simulink model "SimFreqDynamics"  (R2023a)
settings: Solver=VariableStepAuto  StartTime=0.0  StopTime=0.4  RelTol=1e-3
values from neighbouring files (symbols this model uses):
  L = X/Wbase    (= 0.0031194368846)    [ParaFreqVoltageEquivalance.m]
  R = X/5    (= 0.196)    [ParaFreqVoltageEquivalance.m]
  Sbase = 1    [ParaFreqDynamics.m]    (also in ParaFreqVoltageEquivalance.m; SimModel_Parameters.m)
  Ts = 1/Fs    (= 1e-05)    [ParaFreqDynamics.m]    (also in ParaFreqVoltageEquivalance.m; SimModel_Parameters.m = 0.0001)
  Vbase = 1    [ParaFreqDynamics.m]    (also in ParaFreqVoltageEquivalance.m; SimModel_Parameters.m)
  Wbase = Fbase*2*pi    (= 314.159265359)    [ParaFreqDynamics.m]    (also in ParaFreqVoltageEquivalance.m; SimModel_Parameters.m)
undefined symbols (not defined in the file or in its folder): DiscIntNeverNeededParam
libraries: spsCurrentMeasurementLib x6, spsSeriesRLCBranchLib x3, spsControlledVoltageSourceLib x3, spsGroundLib x2, SimplusGT x1, spsThreePhaseSeriesRLCBranchLib x1, sps_lib x1
settings Model: Creator=admin_user  LastModifiedBy=admin_user

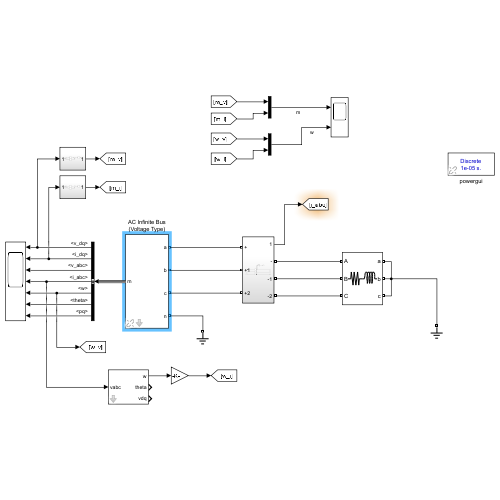
[thumbnail: Simulink's stored preview of the top-level diagram]
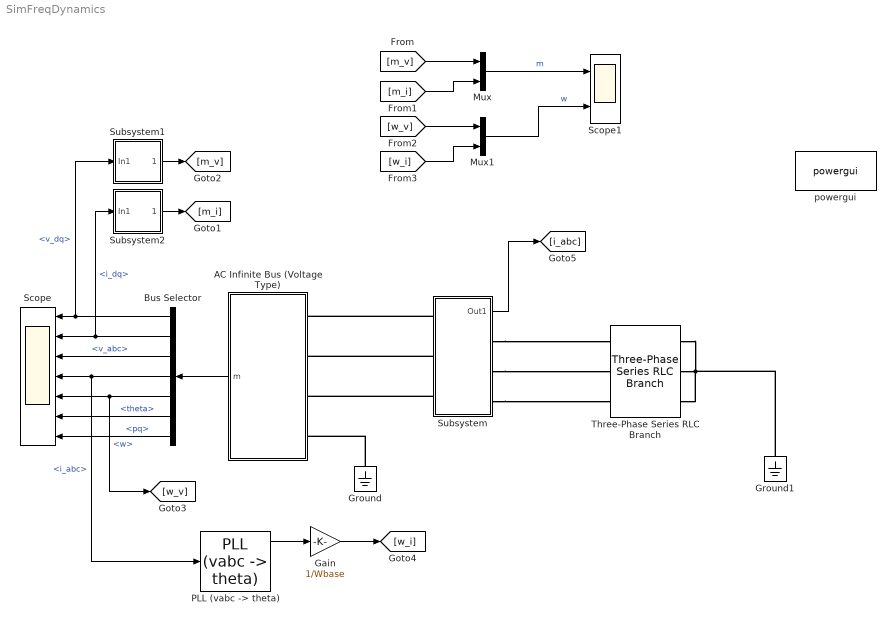
== system SimFreqDynamics ==
  AC Infinite Bus (Voltage Type) : Subsystem  AncestorBlock=|  mask{Ts=Ts, Sbase=Sbase, Vbase=Vbase, Wbase=Wbase, vd=1, vq=0, theta0=0, w=Wbase, R=1e-30}
      | SimplusGT/AC Infinite Bus
      | (Voltage Type)
      mask prompts: Ts "Ts (s), samping period"; Sbase "Sbase (VA), power base"; Vbase "Vbase (V), voltage base"; Wbase "Wbase (rad/s), frequency base"; vd "vd (pu), d-axis voltage"; vq "vq (pu), q-axis voltage"; theta0 "theta0 (rad), initial angle"; w "w (rad/s), frequency"; R "R (Ohm), resistance"
  Bus Selector : BusSelector  OutputSignals=v_dq,i_dq,v_abc,i_abc,w,theta,pq
  Gain : Gain  Gain=1/Wbase
  Ground : spsGroundLib/Ground  LConnTagsString=a
  Ground1 : spsGroundLib/Ground  LConnTagsString=a
  Mux : Mux  Inputs=2
  Mux1 : Mux  Inputs=2
  "PLL (vabc -> theta)" : SimplusGT/PLL (vabc -> theta)  Ts=Ts  Wbase=Wbase  w_pll=w_pll  w_tau=w_tau  theta0=0
      settings: SourceProductName=Simplus Grid Tool
  Scope : Scope  NumInputPorts=7
  Scope1 : Scope  NumInputPorts=2
  Subsystem : Subsystem
  Subsystem1 : Subsystem
  Subsystem2 : Subsystem
  Three-Phase Series RLC Branch : spsThreePhaseSeriesRLCBranchLib/Three-Phase Series RLC Branch  LConnTagsString=A|B|C  RConnTagsString=A|B|C  BranchType=RL  Resistance=R  Inductance=L  Capacitance=1e-6  Measurements=None
  powergui : sps_lib/powergui  Priority=1  SimulationMode=Discrete  SampleTime=Ts  frequency=60  Iterations=50  frequencyindice=0  Pbase=100e6  ErrMax=1e-4  UnitsV=kV  UnitsW=MW  buscounter=0  FunctionMessages=off  echomessages=off  EnableUseOfTLC=off  CurrentSourceSwitches=off  DisableSnubberDevices=off  DisableRonSwitches=off  DisableVfSwitches=off  DisplayEquations=off  AutomaticDiscreteSolvers=off  SolverType=Tustin/Backward Euler (TBE)  Interpol=off  ExternalGateDelay=off  methode=off  Ts=100  x0status=blocks  SPID=on  SwTol=0  HookPort=off  NonlinearTolerance=1e-4  nMaxIteration=100  ContinueOnMaxIteration=off  RestoreLinks=warning  ResistiveCurrentMeasurement=off  Frange=[0:2:500]  Ylog=off  Xlog=on  ShowGrid=off  save=off  variable=ZData  structure=0  ZoomFFT=off  StartTime=0.0  cycles=1  DisplayStyle=1  fundamental=60  FreqAxis=off  MaxFrequency=1000  frequencyindicesteady=1  RmsSteady=1  display=off
  wires:
  AC Infinite Bus (Voltage Type)/1(m) -> Bus Selector/1
  Bus Selector/1 -> Subsystem1/1(In1), Scope/1  "<v_dq>"
  Bus Selector/3 -> Scope/3  "<v_abc>"
  Bus Selector/4 -> "PLL (vabc -> theta)"/1, Scope/4  "<i_abc>"
  Bus Selector/5 -> [w_v], Scope/5  "<w>"
  Bus Selector/6 -> Scope/6  "<theta>"
  Bus Selector/7 -> Scope/7  "<pq>"
  Subsystem/1(Out1) -> [i_abc]
  Subsystem1/1(Out1) -> [m_v]
  Bus Selector/2 -> Scope/2, Subsystem2/1(In1)  "<i_dq>"
  Subsystem2/1(Out1) -> [m_i]
  "PLL (vabc -> theta)"/1 -> Gain/1
  [m_v] -> Mux/1
  [m_i] -> Mux/2
  [w_v] -> Mux1/1
  [w_i] -> Mux1/2
  Mux/1 -> Scope1/1  "m"
  Mux1/1 -> Scope1/2  "w"
  Gain/1 -> [w_i]
  connections:
  Three-Phase Series RLC Branch/RConn1 -- Three-Phase Series RLC Branch/RConn2 -- Three-Phase Series RLC Branch/RConn3 -- Ground1/LConn1
  Ground/LConn1 -- AC Infinite Bus (Voltage Type)/LConn4
  Subsystem/LConn1 -- AC Infinite Bus (Voltage Type)/LConn1
  Subsystem/RConn1 -- Three-Phase Series RLC Branch/LConn1
  Subsystem/LConn2 -- AC Infinite Bus (Voltage Type)/LConn2
  Subsystem/RConn2 -- Three-Phase Series RLC Branch/LConn2
  Subsystem/LConn3 -- AC Infinite Bus (Voltage Type)/LConn3
  Subsystem/RConn3 -- Three-Phase Series RLC Branch/LConn3

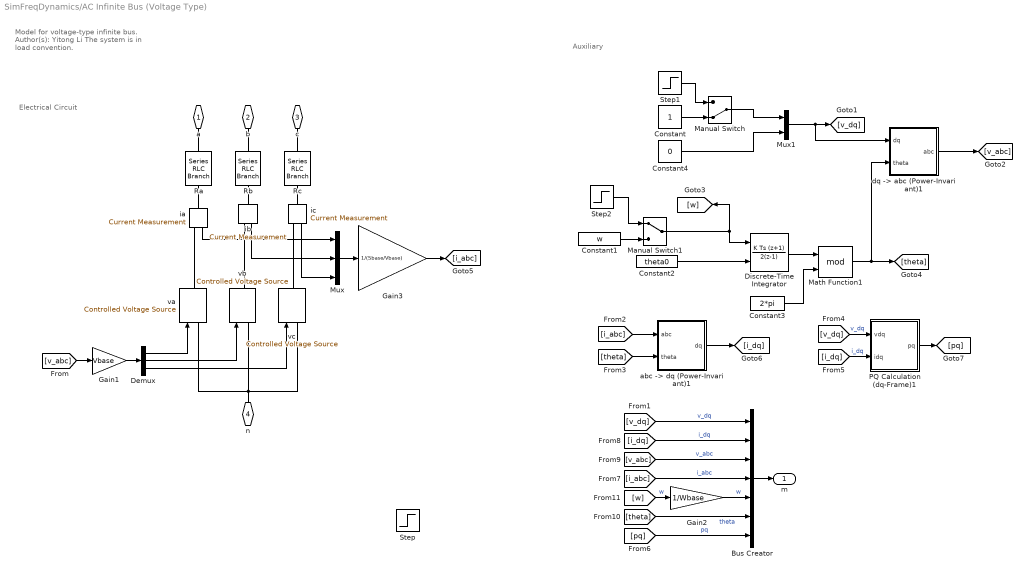
== system SimFreqDynamics/AC Infinite Bus (Voltage Type) ==
  note: Auxiliary
  note: Electrical Circuit
  note: Model for voltage-type infinite bus.
      |
      | Author(s): Yitong Li
      |
      | The system is in load convention.
  Bus Creator : BusCreator  Inputs=7
  Constant : Constant
  Constant1 : Constant  Value=w
  Constant2 : Constant  Value=theta0
  Constant3 : Constant  Value=2*pi
  Constant4 : Constant  Value=0
  Demux : Demux  Outputs=3
  Discrete-Time Integrator : DiscreteIntegrator  IntegratorMethod=Integration: Trapezoidal  InitialConditionSource=external  SampleTime=-1  ICPrevOutput=DiscIntNeverNeededParam  ICPrevScaledInput=DiscIntNeverNeededParam
  Gain1 : Gain  Gain=Vbase
  Gain2 : Gain  Gain=1/Wbase
  Gain3 : Gain  Gain=1/(Sbase/Vbase)
  Manual Switch : ManualSwitch  CurrentSetting=0
  Manual Switch1 : ManualSwitch
  Math Function1 : Math  Operator=mod  SignedPower=on
  Mux : Mux  Inputs=3
  Mux1 : Mux  Inputs=2
  PQ Calculation (dq-Frame)1 : Subsystem  AncestorBlock=|
      | SimplusGT/PQ Calculation
      | (dq-Frame)
  Ra : spsSeriesRLCBranchLib/Series RLC Branch  LConnTagsString=__new0  RConnTagsString=__new0  BranchType=R  Resistance=R  Inductance=1e-3  SetiL0=off  InitialCurrent=0  Capacitance=1e-6  Setx0=off  InitialVoltage=0  Measurements=None
  Rb : spsSeriesRLCBranchLib/Series RLC Branch  LConnTagsString=__new0  RConnTagsString=__new0  BranchType=R  Resistance=R  Inductance=1e-3  SetiL0=off  InitialCurrent=0  Capacitance=1e-6  Setx0=off  InitialVoltage=0  Measurements=None
  Rc : spsSeriesRLCBranchLib/Series RLC Branch  LConnTagsString=__new0  RConnTagsString=__new0  BranchType=R  Resistance=R  Inductance=1e-3  SetiL0=off  InitialCurrent=0  Capacitance=1e-6  Setx0=off  InitialVoltage=0  Measurements=None
  Step : Step  SampleTime=0
  Step1 : Step  Time=0.2  Before=1  After=1.1  SampleTime=0
  Step2 : Step  Time=0.2  Before=1*Wbase  After=1.1*Wbase  SampleTime=0
  "abc -> dq (Power-Invariant)1" : Subsystem  AncestorBlock=|
      | SimplusGT/abc -> dq
      | (Power-Invariant)
  "dq -> abc (Power-Invariant)1" : Subsystem  AncestorBlock=|
      | SimplusGT/dq -> abc
      | (Power-Invariant)
  ia : spsCurrentMeasurementLib/Current Measurement  PhasorSimulation=off  OutputType=Complex  PSBequivalent=0
  ib : spsCurrentMeasurementLib/Current Measurement  PhasorSimulation=off  OutputType=Complex  PSBequivalent=0
  ic : spsCurrentMeasurementLib/Current Measurement  PhasorSimulation=off  OutputType=Complex  PSBequivalent=0
  va : spsControlledVoltageSourceLib/Controlled Voltage Source  Initialize=on  Source_Type=AC  Amplitude=0  Phase=0  Frequency=0  Measurements=None
  vb : spsControlledVoltageSourceLib/Controlled Voltage Source  Initialize=on  Source_Type=AC  Amplitude=0  Phase=0  Frequency=0  Measurements=None
  vc : spsControlledVoltageSourceLib/Controlled Voltage Source  Initialize=on  Source_Type=AC  Amplitude=0  Phase=0  Frequency=0  Measurements=None
  a : PMIOPort  Side=Left
  b : PMIOPort  Port=2  Side=Left
  c : PMIOPort  Port=3  Side=Left
  n : PMIOPort  Port=4  Side=Left
  m : Outport
  wires:
  [pq] -> Bus Creator/7  "pq"
  PQ Calculation (dq-Frame)1/1(pq) -> [pq]
  [i_dq] -> PQ Calculation (dq-Frame)1/2(idq)  "i_dq"
  [v_dq] -> PQ Calculation (dq-Frame)1/1(vdq)  "v_dq"
  Gain3/1 -> [i_abc]
  Mux/1 -> Gain3/1
  Gain1/1 -> Demux/1
  "abc -> dq (Power-Invariant)1"/1(dq) -> [i_dq]
  [theta] -> "abc -> dq (Power-Invariant)1"/2(theta)
  [i_abc] -> "abc -> dq (Power-Invariant)1"/1(abc)
  ic/1 -> Mux/3
  ib/1 -> Mux/2
  ia/1 -> Mux/1
  [theta] -> Bus Creator/6  "theta"
  Bus Creator/1 -> m/1
  [i_dq] -> Bus Creator/2  "i_dq"
  Gain2/1 -> Bus Creator/5  "w"
  [v_abc] -> Bus Creator/3  "v_abc"
  [w] -> Gain2/1  "w"
  [i_abc] -> Bus Creator/4  "i_abc"
  [v_dq] -> Bus Creator/1  "v_dq"
  Discrete-Time Integrator/1 -> Math Function1/1
  Constant3/1 -> Math Function1/2
  "dq -> abc (Power-Invariant)1"/1(abc) -> [v_abc]
  Constant2/1 -> Discrete-Time Integrator/2
  Math Function1/1 -> [theta], "dq -> abc (Power-Invariant)1"/2(theta)
  Demux/3 -> vc/1
  Demux/2 -> vb/1
  Demux/1 -> va/1
  [v_abc] -> Gain1/1
  Constant4/1 -> Mux1/2
  Mux1/1 -> [v_dq], "dq -> abc (Power-Invariant)1"/1(dq)
  Constant/1 -> Manual Switch/2
  Manual Switch/1 -> Mux1/1
  Step1/1 -> Manual Switch/1
  Manual Switch1/1 -> Discrete-Time Integrator/1, [w]
  Constant1/1 -> Manual Switch1/2
  Step2/1 -> Manual Switch1/1
  connections:
  Rc/LConn1 -- c/RConn1
  Rc/RConn1 -- ic/LConn1
  Rb/LConn1 -- b/RConn1
  ib/LConn1 -- Rb/RConn1
  Ra/LConn1 -- a/RConn1
  Ra/RConn1 -- ia/LConn1
  ic/RConn1 -- vc/RConn1
  ib/RConn1 -- vb/RConn1
  ia/RConn1 -- va/RConn1
  vb/LConn1 -- va/LConn1 -- n/RConn1 -- vc/LConn1

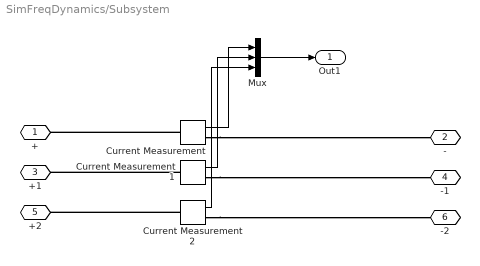
== system SimFreqDynamics/Subsystem ==
  Current Measurement : spsCurrentMeasurementLib/Current Measurement  PhasorSimulation=off  OutputType=Complex  PSBequivalent=0
  Current Measurement1 : spsCurrentMeasurementLib/Current Measurement  PhasorSimulation=off  OutputType=Complex  PSBequivalent=0
  Current Measurement2 : spsCurrentMeasurementLib/Current Measurement  PhasorSimulation=off  OutputType=Complex  PSBequivalent=0
  Mux : Mux  Inputs=3
  + : PMIOPort  Side=Left
  - : PMIOPort  Port=2  Side=Right
  +1 : PMIOPort  Port=3  Side=Left
  -1 : PMIOPort  Port=4  Side=Right
  +2 : PMIOPort  Port=5  Side=Left
  -2 : PMIOPort  Port=6  Side=Right
  Out1 : Outport
  wires:
  Current Measurement2/1 -> Mux/3
  Current Measurement1/1 -> Mux/2
  Current Measurement/1 -> Mux/1
  Mux/1 -> Out1/1
  connections:
  Current Measurement2/RConn1 -- -2/RConn1
  Current Measurement/RConn1 -- -/RConn1
  Current Measurement2/LConn1 -- +2/RConn1
  Current Measurement1/RConn1 -- -1/RConn1
  Current Measurement1/LConn1 -- +1/RConn1
  Current Measurement/LConn1 -- +/RConn1

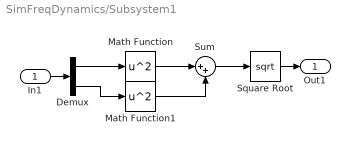
== system SimFreqDynamics/Subsystem1 ==
  In1 : Inport
  Demux : Demux  Outputs=2
  Math Function : Math  Operator=square
  Math Function1 : Math  Operator=square
  Square Root : Sqrt
  Sum : Sum  Inputs=|++
  Out1 : Outport
  wires:
  Math Function1/1 -> Sum/2
  Sum/1 -> Square Root/1
  Demux/1 -> Math Function/1
  Math Function/1 -> Sum/1
  Demux/2 -> Math Function1/1
  Square Root/1 -> Out1/1
  In1/1 -> Demux/1

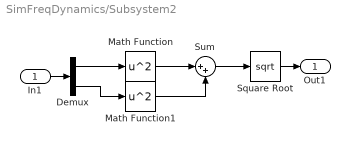
== system SimFreqDynamics/Subsystem2 ==
  In1 : Inport
  Demux : Demux  Outputs=2
  Math Function : Math  Operator=square
  Math Function1 : Math  Operator=square
  Square Root : Sqrt
  Sum : Sum  Inputs=|++
  Out1 : Outport
  wires:
  Math Function1/1 -> Sum/2
  Sum/1 -> Square Root/1
  Demux/1 -> Math Function/1
  Math Function/1 -> Sum/1
  Demux/2 -> Math Function1/1
  Square Root/1 -> Out1/1
  In1/1 -> Demux/1

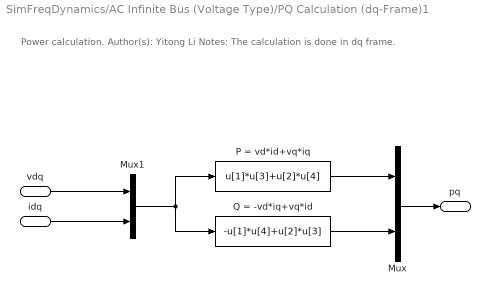
== system SimFreqDynamics/AC Infinite Bus (Voltage Type)/PQ Calculation (dq-Frame)1 ==
  note: Power calculation.
      |
      | Author(s): Yitong Li
      |
      | Notes:
      |
      | The calculation is done in dq frame.
  vdq : Inport
  idq : Inport  Port=2
  Mux : Mux  Inputs=2
  Mux1 : Mux  Inputs=2
  P = vd*id+vq*iq : Fcn  Expr=u[1]*u[3]+u[2]*u[4]
  Q = -vd*iq+vq*id : Fcn  Expr=-u[1]*u[4]+u[2]*u[3]
  pq : Outport
  wires:
  Mux/1 -> pq/1
  P = vd*id+vq*iq/1 -> Mux/1
  vdq/1 -> Mux1/1
  idq/1 -> Mux1/2
  Mux1/1 -> P = vd*id+vq*iq/1, Q = -vd*iq+vq*id/1
  Q = -vd*iq+vq*id/1 -> Mux/2

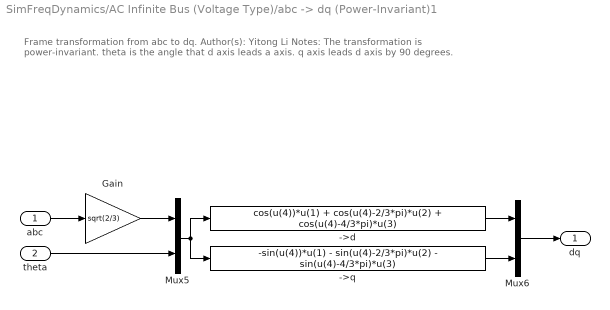
== system SimFreqDynamics/AC Infinite Bus (Voltage Type)/abc -> dq (Power-Invariant)1 ==
  note: Frame transformation from abc to dq.
      |
      | Author(s): Yitong Li
      |
      | Notes:
      |
      | The transformation is power-invariant.
      |
      | theta is the angle that d axis leads a axis.
      |
      | q axis leads d axis by 90 degrees.
  abc : Inport
  theta : Inport  Port=2
  ->d : Fcn  Expr=cos(u(4))*u(1) + cos(u(4)-2/3*pi)*u(2) + cos(u(4)-4/3*pi)*u(3)
  ->q : Fcn  Expr=-sin(u(4))*u(1) - sin(u(4)-2/3*pi)*u(2) - sin(u(4)-4/3*pi)*u(3)
  Gain : Gain  Gain=sqrt(2/3)
  Mux5 : Mux  Inputs=2
  Mux6 : Mux  Inputs=2
  dq : Outport
  wires:
  abc/1 -> Gain/1
  ->d/1 -> Mux6/1
  Gain/1 -> Mux5/1
  theta/1 -> Mux5/2
  ->q/1 -> Mux6/2
  Mux6/1 -> dq/1
  Mux5/1 -> ->d/1, ->q/1

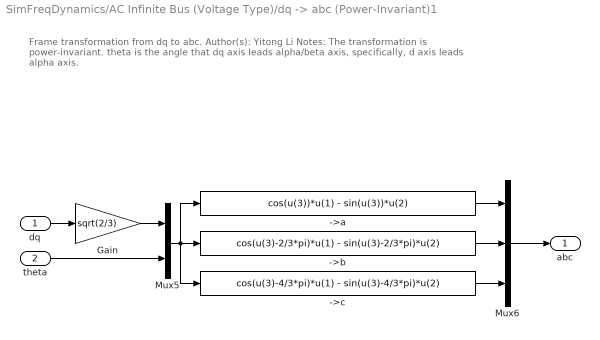
== system SimFreqDynamics/AC Infinite Bus (Voltage Type)/dq -> abc (Power-Invariant)1 ==
  note: Frame transformation from dq to abc.
      |
      | Author(s): Yitong Li
      |
      | Notes:
      |
      | The transformation is power-invariant.
      |
      | theta is the angle that dq axis leads alpha/beta axis, specifically, d axis leads alpha axis.
  dq : Inport
  theta : Inport  Port=2
  ->a : Fcn  Expr=cos(u(3))*u(1) - sin(u(3))*u(2)
  ->b : Fcn  Expr=cos(u(3)-2/3*pi)*u(1) - sin(u(3)-2/3*pi)*u(2)
  ->c : Fcn  Expr=cos(u(3)-4/3*pi)*u(1) - sin(u(3)-4/3*pi)*u(2)
  Gain : Gain  Gain=sqrt(2/3)
  Mux5 : Mux  Inputs=2
  Mux6 : Mux  Inputs=3
  abc : Outport
  wires:
  ->b/1 -> Mux6/2
  ->a/1 -> Mux6/1
  Gain/1 -> Mux5/1
  dq/1 -> Gain/1
  ->c/1 -> Mux6/3
  Mux6/1 -> abc/1
  Mux5/1 -> ->b/1, ->a/1, ->c/1
  theta/1 -> Mux5/2
